simulink model "sbv"  (R2012b)
settings: Solver=ode45  StartTime=0.0  StopTime=10.0  RelTol=1e-3
settings Model: Creator=Administrator  LastModifiedBy=Administrator

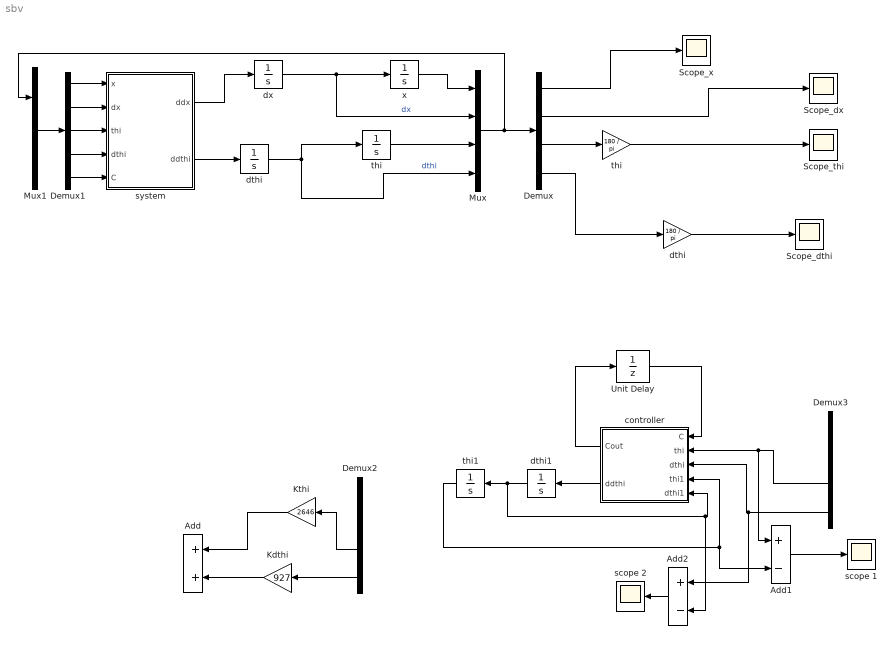
== system sbv ==
  Add : Sum
  Add1 : Sum  Inputs=+-
  Add2 : Sum  Inputs=+-
  Demux : Demux
  Demux1 : Demux  Outputs=5
  Demux2 : Demux
  Demux3 : Demux
  Kdthi : Gain  Gain=927
  Kthi : Gain  Gain=2646
  Mux : Mux
  Mux1 : Mux  Inputs=2
  Scope_dthi : Scope
      settings: SaveName=ScopeData3
  Scope_dx : Scope
  Scope_thi : Scope
      settings: SaveName=ScopeData2
  Scope_x : Scope
  Unit Delay : UnitDelay  SampleTime=-1
  controller : MATLAB Function  TreatAsAtomicUnit=on
  dthi : Integrator
  "dthi " : Gain  Gain=180 / pi
  dthi1 : Integrator
  dx : Integrator
  scope 1 : Scope
      settings: SaveName=ScopeData5
  scope 2 : Scope
      settings: SaveName=ScopeData4
  system : MATLAB Function  TreatAsAtomicUnit=on
  thi : Integrator  InitialCondition=15 * pi / 180
  "thi " : Gain  Gain=180 / pi
  thi1 : Integrator
  x : Integrator
  wires:
  system/1(ddx) -> dx/1
  dx/1 -> Mux/2, x/1  "dx"
  system/2(ddthi) -> dthi/1
  dthi/1 -> Mux/4, thi/1  "dthi"
  x/1 -> Mux/1
  thi/1 -> Mux/3
  Mux/1 -> Demux/1, Mux1/1
  Demux1/5 -> system/5(C)
  Demux1/4 -> system/4(dthi)
  Demux1/3 -> system/3(thi)
  Demux1/2 -> system/2(dx)
  Demux1/1 -> system/1(x)
  Mux1/1 -> Demux1/1
  Kthi/1 -> Add/1
  Kdthi/1 -> Add/2
  Demux2/3 -> Kthi/1
  Demux2/4 -> Kdthi/1
  Demux/3 -> "thi "/1
  Demux/4 -> "dthi "/1
  Demux/1 -> Scope_x/1
  Demux/2 -> Scope_dx/1
  "thi "/1 -> Scope_thi/1
  "dthi "/1 -> Scope_dthi/1
  controller/2(ddthi) -> dthi1/1
  dthi1/1 -> Add2/2, controller/5(dthi1), thi1/1
  controller/1(Cout) -> Unit Delay/1
  Demux3/3 -> Add1/1, controller/2(thi)
  Demux3/4 -> Add2/1, controller/3(dthi)
  Unit Delay/1 -> controller/1(C)
  thi1/1 -> Add1/2, controller/4(thi1)
  Add1/1 -> scope 1/1
  Add2/1 -> scope 2/1

== matlab function sbv/controller ==
  data: C input; thi input; dthi input; thi1 input; dthi1 input; Cout output; ddthi output
function [Cout, ddthi] = fcn(C, thi, dthi, thi1, dthi1)
Mp = 135;
Mr = 5.5;
D = 0.6;
L = 1;
b = 0.03;
R = 0.2;
Jp = 27.6;
Jr = 0.11;
g = 9.8;

%**************************************************************************
%线性模型
%**************************************************************************
alpha = Mr * R ^ 2 / Jr + 1;
beta = Jp / (Mp * L) + L;
gama = L * Mp * g;
A22 = -R ^ 2 * b / (alpha * Jr);
A23 = -R ^ 2 * gama / (2 * Jr * alpha * beta);
B2 = R / (2 * Jr) * (1 / alpha + R / (alpha * beta));
A43 = gama / Jp - (L * gama) / (Jp * beta);
B4 = (L / beta - 1) / Jp;
%**************************************************************************
%dthi = dthi + 1227400 * (thi - thi1) + 430300 * (dthi - dthi1);
ddthi = A43 * thi + B4 * C + 430300 * (thi - thi1) + 150800 * (dthi - dthi1);
Cout = 2646 * thi1 + 927 * dthi1;

== matlab function sbv/system ==
  data: x input; ddx output; dx input; thi input; dthi input; C input; ddthi output
function [ddx,ddthi] = fcn(x,dx,thi,dthi,C)
Mp = 200;
Mr = 5.5;
D = 0.6;
L = 1;
b = 0.03;
R = 0.2;
Jp = 27.6;
Jr = 0.11;
g = 9.8;

%**************************************************************************
%非线性模型
%**************************************************************************
alpha = Mr * R ^ 2 / Jr + 1;
beta = Jp / (Mp * L * cos(thi)) + L * cos(thi);
gama = L * Mp * g;
A22 = -R ^ 2 * b / (alpha * Jr);
A23 = -R ^ 2 * (gama - Jp * dthi ^ 2 / cos(thi)) / (2 * Jr * alpha * beta);
B2 = R / (2 * Jr) * (1 / alpha + R / (alpha * beta));
A43 = gama / Jp - (L * (gama * cos(thi) - Jp * dthi ^ 2) / (Jp * beta));
B4 = (L * cos(thi) / beta - 1) / Jp;

f2 = 0;
f4 = 0;

ddx = A22 * dx + A23 * sin(thi) + B2 * C + f2;
ddthi = A43 * sin(thi) + B4 * C + f4;

% %**************************************************************************
% %线性模型
% %**************************************************************************
% alpha = Mr * R ^ 2 / Jr + 1;
% beta = Jp / (Mp * L) + L;
% gama = L * Mp * g;
% A22 = -R ^ 2 * b / (alpha * Jr);
% A23 = -R ^ 2 * gama / (2 * Jr * alpha * beta);
% B2 = R / (2 * Jr) * (1 / alpha + R / (alpha * beta));
% A43 = gama / Jp - (L * gama) / (Jp * beta);
% B4 = (L / beta - 1) / Jp;
% 
% ddx = A22 * dx + A23 * thi + B2 * C;% + wgn(1, 1, 0);
% ddthi = A43 * thi + B4 * C;% + wgn(1, 1, 0);
% %**************************************************************************
